simulink model "M_T_simu"  (R2024a)
settings: Solver=VariableStepAuto  StartTime=0.0  StopTime=5  RelTol=1e-3
values from neighbouring files (symbols this model uses):
  b1 = 1000    [M_T.m]    (also in Parameters_m_t.m)
  k1 = 16182    [M_T.m]    (also in Parameters_m_t.m)
  k2 = 19000    [M_T.m]    (also in Parameters_m_t.m)
  m1 = 290    [M_T.m]    (also in Parameters_m_t.m)
  m2 = 59    [M_T.m]    (also in Parameters_m_t.m)
settings Model: Creator=Aguirre  LastModifiedBy=Aguirre

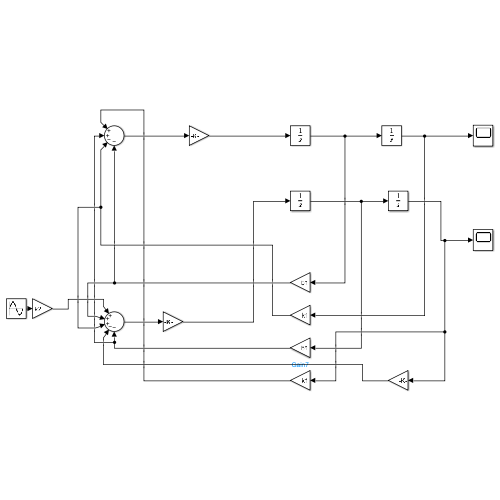
[thumbnail: Simulink's stored preview of the top-level diagram]
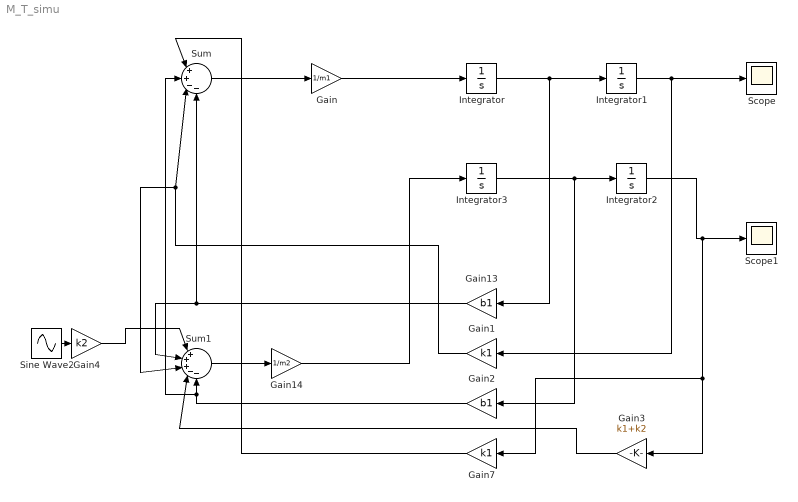
== system M_T_simu ==
  Gain : Gain  Gain=1/m1
  Gain1 : Gain  Gain=k1
  Gain13 : Gain  Gain=b1
  Gain14 : Gain  Gain=1/m2
  Gain2 : Gain  Gain=b1
  Gain3 : Gain  Gain=k1+k2
  Gain4 : Gain  Gain=k2
  Gain7 : Gain  Gain=k1
  Integrator{,1..3} (4 alike) : Integrator
  Scope : Scope
  Scope1 : Scope
  Sine Wave2 : Sin  Amplitude=0.05  Frequency=20*pi  SampleTime=0
  Sum : Sum  Inputs=|++--
  Sum1 : Sum  Inputs=|+++--
  wires:
  Sum/1 -> Gain/1
  Gain/1 -> Integrator/1
  Integrator/1 -> Gain13/1, Integrator1/1
  Gain14/1 -> Integrator3/1
  Integrator3/1 -> Gain2/1, Integrator2/1
  Integrator1/1 -> Scope/1, Gain1/1
  Integrator2/1 -> Gain7/1, Gain3/1, Scope1/1
  Sum1/1 -> Gain14/1
  Sine Wave2/1 -> Gain4/1
  Gain4/1 -> Sum1/1
  Gain13/1 -> Sum1/2, Sum/4
  Gain1/1 -> Sum1/3, Sum/3
  Gain2/1 -> Sum/2, Sum1/5
  Gain7/1 -> Sum/1
  Gain3/1 -> Sum1/4
